simulink model "CACC_4_Robots_Example_Cases"  (R2021a)
settings: Solver=FixedStepAuto  StartTime=0.0  StopTime=Tsim  RelTol=1e-3
values from neighbouring files (symbols this model uses):
  cIN = 0    [ros_cacc.m]    (also in ros_cacc2.m = 4)
  h = 1.0    (= 1)    [ros_cacc.m]    (also in ros_cacc2.m)
  k1 = 1    [ros_cacc.m]    (also in ros_cacc2.m)
  k2 = 1    [ros_cacc.m]    (also in ros_cacc2.m)
  r = 1    [ros_cacc.m]    (also in ros_cacc2.m)
  v_0 = 0.5    [ros_cacc.m]    (also in ros_cacc2.m)
  v_threshold = v_thr    (= 0.1)    [ros_cacc.m]    (also in ros_cacc2.m)
undefined symbols (not defined in the file or in its folder): angular, linear, sigbuilder_block
libraries: ros2lib x23, robotcorelib x4
(part 1 of 3)
settings Model: Creator=harun  LastModifiedBy=harun
settings DataIOCC: DSMLogging=off  ReturnWorkspaceOutputs=off
settings OptimizationCC: EnhancedBackFolding=on  PassReuseOutputArgsAs=Individual arguments  ZeroExternalMemoryAtStartup=off  ZeroInternalMemoryAtStartup=off  MaxStackSize=64  OptimizeBlockOrder=speed  DifferentSizesBufferReuse=on  OptimizationCustomize=off  EfficientTunableParamExpr=on
settings DebuggingCC: ParameterTunabilityLossMsg=error
settings HardwareCC: ProdBitPerLong=64  ProdHWDeviceType=AMD->x86-64 (Linux 64)
settings SFSimCC: MATLABDynamicMemAlloc=off
settings RTWCC: SystemTargetFile=ert.tlc  HardwareBoard=Robot Operating System 2 (ROS 2)  TemplateMakefile=ert_default_tmf  Toolchain=Colcon Tools  TargetLang=C++
settings CodeAppCC: ForceParamTrailComments=on  IgnoreCustomStorageClasses=off  OperatorAnnotations=on  SimulinkDataObjDesc=on  SFDataObjDesc=on  InsertBlockDesc=on
settings ERTTargetCC: CodeInterfacePackaging=C++ class  SupportContinuousTime=on  SupportVariableSizeSignals=on  RootIOFormat=Structure reference

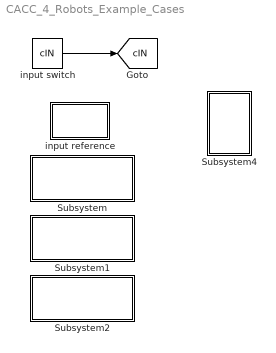
== system CACC_4_Robots_Example_Cases ==
  Subsystem : Subsystem
  Subsystem1 : Subsystem
  Subsystem2 : Subsystem
  Subsystem4 : Subsystem
  input reference : Subsystem
  input switch : Constant  Value=cIN
  tag scope: cIN=global
  wires:
  input switch/1 -> [cIN]

== system CACC_4_Robots_Example_Cases/Subsystem ==
  Bus Creator : BusCreator  Inputs=2
  Terminator : Terminator
  Terminator1 : Terminator
  To Workspace : ToWorkspace  VariableName=robot1  SaveFormat=Timeseries  SampleTime=-1
  To Workspace1 : ToWorkspace  VariableName=robot1input  SaveFormat=Timeseries  SampleTime=0.01
  controllers : Subsystem
  subscriber : Subsystem
  vehicle w/o CACC : Subsystem
  wires:
  controllers/2(z) -> Terminator/1
  vehicle w/o CACC/1(state) -> Bus Creator/1, controllers/2(state)
  controllers/1(a,w) -> vehicle w/o CACC/1(a,w)
  controllers/3(xLA,yLA) -> Bus Creator/2, Terminator1/1
  Bus Creator/1 -> To Workspace/1
  subscriber/1(state) -> To Workspace1/1, vehicle w/o CACC/2(v), controllers/1(state_prec)

== system CACC_4_Robots_Example_Cases/Subsystem1 ==
  Bus Creator : BusCreator  Inputs=2
  Terminator : Terminator
  Terminator1 : Terminator
  To Workspace : ToWorkspace  VariableName=robot2  SaveFormat=Timeseries  SampleTime=-1
  controllers : Subsystem
  subscriber : Subsystem
  vehicle w/o CACC : Subsystem
  wires:
  subscriber/1(state1) -> vehicle w/o CACC/2(v), controllers/1(state_prec)
  controllers/2(z) -> Terminator/1
  controllers/1(a,w) -> vehicle w/o CACC/1(a,w)
  vehicle w/o CACC/1(state) -> Bus Creator/1, controllers/2(state)
  controllers/3(xLA,yLA) -> Bus Creator/2, Terminator1/1
  Bus Creator/1 -> To Workspace/1

== system CACC_4_Robots_Example_Cases/Subsystem2 ==
  Bus Creator : BusCreator  Inputs=2
  Terminator : Terminator
  Terminator1 : Terminator
  To Workspace : ToWorkspace  VariableName=robot3  SaveFormat=Timeseries  SampleTime=-1
  controllers : Subsystem
  subscriber : Subsystem
  vehicle w/o CACC : Subsystem
  wires:
  subscriber/1(state) -> vehicle w/o CACC/2(v), controllers/1(state_prec)
  controllers/2(z) -> Terminator/1
  controllers/1(a,w) -> vehicle w/o CACC/1(a,w)
  vehicle w/o CACC/1(state) -> Bus Creator/1, controllers/2(state)
  controllers/3(xLA,yLA) -> Bus Creator/2, Terminator1/1
  Bus Creator/1 -> To Workspace/1

== system CACC_4_Robots_Example_Cases/Subsystem4 ==
  Subsystem3 : Subsystem
  To Workspace : ToWorkspace  VariableName=robot0  SaveFormat=Timeseries  SampleTime=-1
  wires:
  Subsystem3/1(state) -> To Workspace/1

== system CACC_4_Robots_Example_Cases/input reference ==
  Switch Case : SwitchCase  CaseConditions={1,2,3}  ShowDefaultCase=off
  circular path small curv : Subsystem  TreatAsAtomicUnit=on
  "circular path, varying velocity" : Subsystem  TreatAsAtomicUnit=on
  random path : Subsystem  TreatAsAtomicUnit=on
  wires:
  Switch Case/2 -> "circular path, varying velocity"/Action
  Switch Case/1 -> circular path small curv/Action
  [cIN] -> Switch Case/1
  Switch Case/3 -> random path/Action

== system CACC_4_Robots_Example_Cases/Subsystem/controllers ==
  state_prec : Inport
  state : Inport  Port=2
  Switch Case Ext. LA : Subsystem  TreatAsAtomicUnit=on
  a,w : Outport  VectorParamsAs1DForOutWhenUnconnected=off
  z : Outport  Port=2  VectorParamsAs1DForOutWhenUnconnected=off
  xLA,yLA : Outport  Port=3  VectorParamsAs1DForOutWhenUnconnected=off
  wires:
  state_prec/1 -> Switch Case Ext. LA/1(state_prec)
  state/1 -> Switch Case Ext. LA/2(state)
  Switch Case Ext. LA/1(a,w) -> a,w/1
  Switch Case Ext. LA/2(z) -> z/1
  Switch Case Ext. LA/3(lookahead point) -> xLA,yLA/1

== system CACC_4_Robots_Example_Cases/Subsystem/subscriber ==
  Bus Creator : BusCreator  Inputs=7
  Bus Selector : BusSelector  OutputSignals=x,y,v,vdot,theta,thetadot
  Derivative2 : Derivative
  Divide : Product  Inputs=*/
  One : Constant  OutDataTypeStr=Inherit: Inherit via back propagation
  Subscribe : ros2lib/Subscribe  topicSource=Specify your own  topic=/robot1/caccCam  messageType=ros_its_msgs/CAM  sampleTime=0.1  QOSHistory=Keep last  QOSDepth=1  QOSReliability=Reliable  QOSDurability=Volatile
      settings: SourceProductBaseCode=RR
  Switch : Switch  Criteria=u2 ~= 0
  Terminator : Terminator
  Terminator4 : Terminator
  state : Outport  VectorParamsAs1DForOutWhenUnconnected=off
  wires:
  Subscribe/1 -> Terminator/1
  Subscribe/2 -> Bus Selector/1
  Bus Selector/4 -> Terminator4/1  "<vdot>"
  One/1 -> Switch/3
  Bus Selector/1 -> Bus Creator/1  "<x>"
  Bus Selector/2 -> Bus Creator/2  "<y>"
  Derivative2/1 -> Bus Creator/4  "vdot"
  Bus Selector/5 -> Bus Creator/5  "<theta>"
  Divide/1 -> Bus Creator/7  "curv"
  Bus Selector/3 -> Bus Creator/3, Derivative2/1, Switch/2, Switch/1  "<v>"
  Bus Creator/1 -> state/1
  Switch/1 -> Divide/2
  Bus Selector/6 -> Divide/1, Bus Creator/6  "<thetadot>"

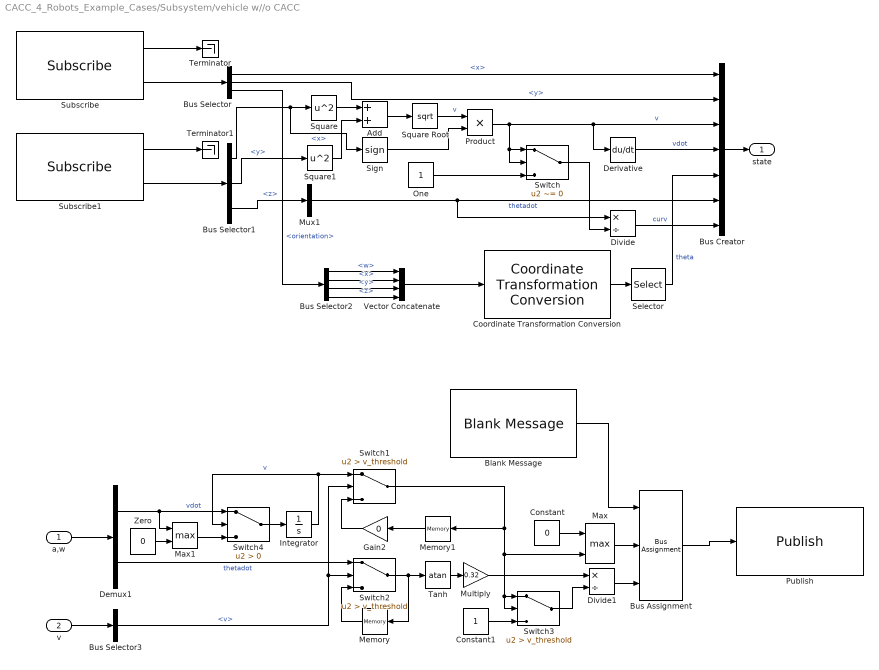
== system CACC_4_Robots_Example_Cases/Subsystem/vehicle w//o CACC ==
  a,w : Inport
  v : Inport  Port=2
  Add : Sum
  Blank Message : ros2lib/Blank Message  messageType=geometry_msgs/Twist  SampleTime=0.01
      settings: SourceProductBaseCode=RR
  Bus Assignment : BusAssignment  AssignedSignals=linear.x,angular.z
  Bus Creator : BusCreator  Inputs=7
  Bus Selector : BusSelector  OutputSignals=pose.position.x,pose.position.y,pose.orientation
  Bus Selector1 : BusSelector  OutputSignals=twist.twist.linear.x,twist.twist.linear.y,twist.twist.angular.z
  Bus Selector2 : BusSelector  OutputSignals=w,x,y,z
  Bus Selector3 : BusSelector  OutputSignals=v
  Constant : Constant  Value=0
  Constant1 : Constant
  Coordinate Transformation Conversion : robotcorelib/Coordinate Transformation Conversion  InputRepresentation=Quaternion  InputEulerSequence=ZYX  ShowTrVecInputPort=on  OutputRepresentation=Euler Angles  OutputEulerSequence=ZYX  ShowTrVecOutputPort=on  SimulateUsing=Interpreted execution
      settings: SourceProductBaseCode=NV,RO,RR,UV
  Demux1 : Demux  Outputs=2
  Derivative : Derivative
  Divide : Product  Inputs=*/
  Divide1 : Product  Inputs=*/
  Gain2 : Gain  Gain=0
  Integrator : Integrator  InitialCondition=v_0
  Max : MinMax  Function=max  Inputs=2
  Max1 : MinMax  Function=max  Inputs=2
  Memory : Memory
  Memory1 : Memory
  Multiply : Gain  Gain=0.32
  Mux1 : Mux  Inputs=1
  One : Constant  OutDataTypeStr=Inherit: Inherit via back propagation
  Product : Product
  Publish : ros2lib/Publish  topicSource=Specify your own  topic=/robot1/cmd_vel  messageType=geometry_msgs/Twist  QOSHistory=Keep last  QOSDepth=1  QOSReliability=Reliable  QOSDurability=Volatile
      settings: SourceProductBaseCode=RR
  Selector : Selector  InputPortWidth=3  IndexOptions=Index vector (dialog)  Indices=[1]  OutputSizes=1
  Sign : Signum
  Square : Math  Operator=square  SaturateOnIntegerOverflow=on
  Square Root : Sqrt  SaturateOnIntegerOverflow=on
  Square1 : Math  Operator=square  SaturateOnIntegerOverflow=on
  Subscribe : ros2lib/Subscribe  topicSource=Specify your own  topic=/robot1/robot_pose  messageType=geometry_msgs/PoseStamped  sampleTime=0.01  QOSHistory=Keep last  QOSDepth=1  QOSReliability=Reliable  QOSDurability=Volatile
      settings: SourceProductBaseCode=RR
  Subscribe1 : ros2lib/Subscribe  topicSource=Specify your own  topic=/robot1/odom  messageType=nav_msgs/Odometry  sampleTime=0.01  QOSHistory=Keep last  QOSDepth=1  QOSReliability=Reliable  QOSDurability=Volatile
      settings: SourceProductBaseCode=RR
  Switch : Switch  Criteria=u2 ~= 0
  Switch1 : Switch  Criteria=u2 > Threshold  Threshold=v_threshold
  Switch2 : Switch  Criteria=u2 > Threshold  Threshold=v_threshold
  Switch3 : Switch  Criteria=u2 > Threshold  Threshold=v_threshold
  Switch4 : Switch  Criteria=u2 > Threshold
  Tanh : Trigonometry  Operator=atan
  Terminator : Terminator
  Terminator1 : Terminator
  Vector Concatenate : Concatenate  NumInputs=4
  Zero : Constant  Value=0  OutDataTypeStr=Inherit: Inherit via back propagation
  state : Outport  VectorParamsAs1DForOutWhenUnconnected=off
  wires:
  Zero/1 -> Max1/2
  Add/1 -> Square Root/1
  Subscribe/1 -> Terminator/1
  Bus Selector1/1 -> Sign/1, Square/1  "<x>"
  a,w/1 -> Demux1/1
  Switch2/1 -> Memory/1, Tanh/1
  Constant/1 -> Max/1
  Bus Selector/2 -> Bus Creator/2  "<y>"
  Bus Selector3/1 -> Switch2/2, Switch1/2  "<v>"
  Bus Selector2/3 -> Vector Concatenate/3  "<y>"
  Bus Assignment/1 -> Publish/1
  Mux1/1 -> Divide/1, Bus Creator/6  "thetadot"
  Memory1/1 -> Gain2/1
  Switch/1 -> Divide/2
  Bus Creator/1 -> state/1
  Tanh/1 -> Multiply/1
  Subscribe1/1 -> Terminator1/1
  Max/1 -> Bus Assignment/2
  Demux1/2 -> Switch2/1  "thetadot"
  Product/1 -> Switch/1, Switch/2, Derivative/1, Bus Creator/3  "v"
  Sign/1 -> Product/2
  Bus Selector2/2 -> Vector Concatenate/2  "<x>"
  Subscribe/2 -> Bus Selector/1
  Selector/1 -> Bus Creator/5  "theta"
  Divide1/1 -> Bus Assignment/3
  Subscribe1/2 -> Bus Selector1/1
  Square1/1 -> Add/2
  Max1/1 -> Switch4/3
  v/1 -> Bus Selector3/1
  Switch1/1 -> Switch3/2, Switch3/1, Max/2, Memory1/1
  Constant1/1 -> Switch3/3
  Bus Selector1/3 -> Mux1/1  "<z>"
  Bus Selector/1 -> Bus Creator/1  "<x>"
  Divide/1 -> Bus Creator/7  "curv"
  Vector Concatenate/1 -> Coordinate Transformation Conversion/1
  Multiply/1 -> Divide1/1
  Bus Selector1/2 -> Square1/1  "<y>"
  Blank Message/1 -> Bus Assignment/1
  Derivative/1 -> Bus Creator/4  "vdot"
  Integrator/1 -> Switch4/2, Switch1/1  "v"
  Demux1/1 -> Max1/1, Switch4/1  "vdot"
  Square Root/1 -> Product/1  "v"
  Switch3/1 -> Divide1/2
  Coordinate Transformation Conversion/1 -> Selector/1
  Square/1 -> Add/1
  One/1 -> Switch/3
  Switch4/1 -> Integrator/1
  Bus Selector/3 -> Bus Selector2/1  "<orientation>"
  Bus Selector2/4 -> Vector Concatenate/4  "<z>"
  Bus Selector2/1 -> Vector Concatenate/1  "<w>"
  Gain2/1 -> Switch1/3
  Memory/1 -> Switch2/3

== system CACC_4_Robots_Example_Cases/Subsystem1/controllers ==
  state_prec : Inport
  state : Inport  Port=2
  Switch Case Ext. LA : Subsystem  TreatAsAtomicUnit=on
  a,w : Outport  VectorParamsAs1DForOutWhenUnconnected=off
  z : Outport  Port=2  VectorParamsAs1DForOutWhenUnconnected=off
  xLA,yLA : Outport  Port=3  VectorParamsAs1DForOutWhenUnconnected=off
  wires:
  state_prec/1 -> Switch Case Ext. LA/1(state_prec)
  state/1 -> Switch Case Ext. LA/2(state)
  Switch Case Ext. LA/1(a,w) -> a,w/1
  Switch Case Ext. LA/2(z) -> z/1
  Switch Case Ext. LA/3(lookahead point) -> xLA,yLA/1

== system CACC_4_Robots_Example_Cases/Subsystem1/subscriber ==
  Bus Creator1 : BusCreator  Inputs=7
  Bus Selector1 : BusSelector  OutputSignals=x,y,v,vdot,theta,thetadot
  Derivative2 : Derivative
  Divide1 : Product  Inputs=*/
  One1 : Constant  OutDataTypeStr=Inherit: Inherit via back propagation
  Subscribe : ros2lib/Subscribe  topicSource=Specify your own  topic=/robot2/caccCam  messageType=ros_its_msgs/CAM  sampleTime=0.1  QOSHistory=Keep last  QOSDepth=1  QOSReliability=Reliable  QOSDurability=Volatile
      settings: SourceProductBaseCode=RR
  Switch1 : Switch  Criteria=u2 ~= 0
  Terminator : Terminator
  Terminator4 : Terminator
  state1 : Outport  VectorParamsAs1DForOutWhenUnconnected=off
  wires:
  Subscribe/1 -> Terminator/1
  Subscribe/2 -> Bus Selector1/1
  Bus Selector1/4 -> Terminator4/1  "<vdot>"
  One1/1 -> Switch1/3
  Bus Selector1/1 -> Bus Creator1/1  "<x>"
  Bus Selector1/2 -> Bus Creator1/2  "<y>"
  Derivative2/1 -> Bus Creator1/4  "vdot"
  Bus Selector1/5 -> Bus Creator1/5  "<theta>"
  Divide1/1 -> Bus Creator1/7  "curv"
  Bus Selector1/3 -> Bus Creator1/3, Derivative2/1, Switch1/2, Switch1/1  "<v>"
  Bus Creator1/1 -> state1/1
  Switch1/1 -> Divide1/2
  Bus Selector1/6 -> Divide1/1, Bus Creator1/6  "<thetadot>"

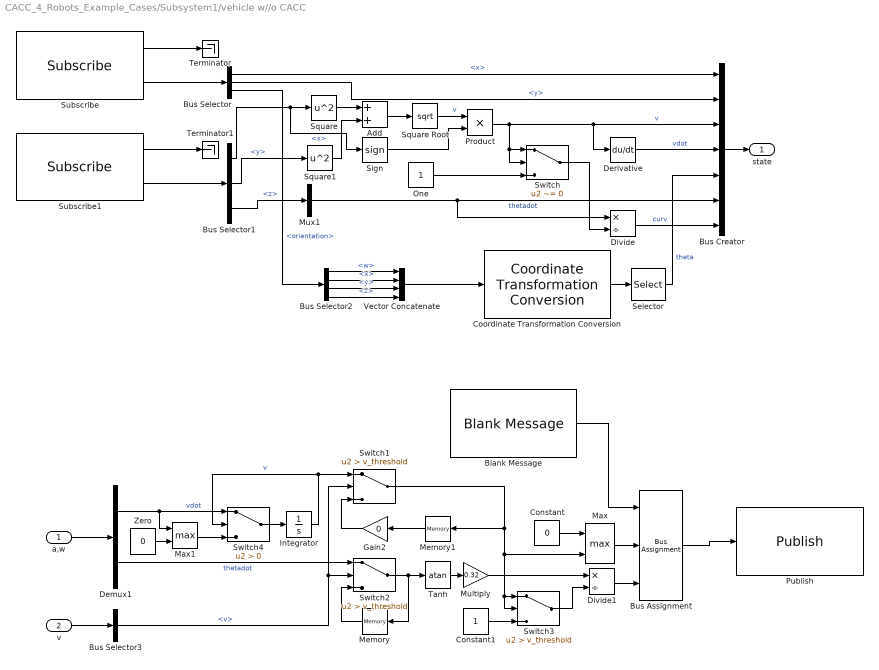
== system CACC_4_Robots_Example_Cases/Subsystem1/vehicle w//o CACC ==
  a,w : Inport
  v : Inport  Port=2
  Add : Sum
  Blank Message : ros2lib/Blank Message  messageType=geometry_msgs/Twist  SampleTime=0.01
      settings: SourceProductBaseCode=RR
  Bus Assignment : BusAssignment  AssignedSignals=linear.x,angular.z
  Bus Creator : BusCreator  Inputs=7
  Bus Selector : BusSelector  OutputSignals=pose.position.x,pose.position.y,pose.orientation
  Bus Selector1 : BusSelector  OutputSignals=twist.twist.linear.x,twist.twist.linear.y,twist.twist.angular.z
  Bus Selector2 : BusSelector  OutputSignals=w,x,y,z
  Bus Selector3 : BusSelector  OutputSignals=v
  Constant : Constant  Value=0
  Constant1 : Constant
  Coordinate Transformation Conversion : robotcorelib/Coordinate Transformation Conversion  InputRepresentation=Quaternion  InputEulerSequence=ZYX  ShowTrVecInputPort=on  OutputRepresentation=Euler Angles  OutputEulerSequence=ZYX  ShowTrVecOutputPort=on  SimulateUsing=Interpreted execution
      settings: SourceProductBaseCode=NV,RO,RR,UV
  Demux1 : Demux  Outputs=2
  Derivative : Derivative
  Divide : Product  Inputs=*/
  Divide1 : Product  Inputs=*/
  Gain2 : Gain  Gain=0
  Integrator : Integrator  InitialCondition=v_0
  Max : MinMax  Function=max  Inputs=2
  Max1 : MinMax  Function=max  Inputs=2
  Memory : Memory
  Memory1 : Memory
  Multiply : Gain  Gain=0.32
  Mux1 : Mux  Inputs=1
  One : Constant  OutDataTypeStr=Inherit: Inherit via back propagation
  Product : Product
  Publish : ros2lib/Publish  topicSource=Specify your own  topic=/robot2/cmd_vel  messageType=geometry_msgs/Twist  QOSHistory=Keep last  QOSDepth=1  QOSReliability=Reliable  QOSDurability=Volatile
      settings: SourceProductBaseCode=RR
  Selector : Selector  InputPortWidth=3  IndexOptions=Index vector (dialog)  Indices=[1]  OutputSizes=1
  Sign : Signum
  Square : Math  Operator=square  SaturateOnIntegerOverflow=on
  Square Root : Sqrt  SaturateOnIntegerOverflow=on
  Square1 : Math  Operator=square  SaturateOnIntegerOverflow=on
  Subscribe : ros2lib/Subscribe  topicSource=Specify your own  topic=/robot2/robot_pose  messageType=geometry_msgs/PoseStamped  sampleTime=0.01  QOSHistory=Keep last  QOSDepth=1  QOSReliability=Reliable  QOSDurability=Volatile
      settings: SourceProductBaseCode=RR
  Subscribe1 : ros2lib/Subscribe  topicSource=Specify your own  topic=/robot2/odom  messageType=nav_msgs/Odometry  sampleTime=0.01  QOSHistory=Keep last  QOSDepth=1  QOSReliability=Reliable  QOSDurability=Volatile
      settings: SourceProductBaseCode=RR
  Switch : Switch  Criteria=u2 ~= 0
  Switch1 : Switch  Criteria=u2 > Threshold  Threshold=v_threshold
  Switch2 : Switch  Criteria=u2 > Threshold  Threshold=v_threshold
  Switch3 : Switch  Criteria=u2 > Threshold  Threshold=v_threshold
  Switch4 : Switch  Criteria=u2 > Threshold
  Tanh : Trigonometry  Operator=atan
  Terminator : Terminator
  Terminator1 : Terminator
  Vector Concatenate : Concatenate  NumInputs=4
  Zero : Constant  Value=0  OutDataTypeStr=Inherit: Inherit via back propagation
  state : Outport  VectorParamsAs1DForOutWhenUnconnected=off
  wires:
  Zero/1 -> Max1/2
  Add/1 -> Square Root/1
  Subscribe/1 -> Terminator/1
  Bus Selector1/1 -> Sign/1, Square/1  "<x>"
  a,w/1 -> Demux1/1
  Switch2/1 -> Memory/1, Tanh/1
  Constant/1 -> Max/1
  Bus Selector/2 -> Bus Creator/2  "<y>"
  Bus Selector3/1 -> Switch2/2, Switch1/2  "<v>"
  Bus Selector2/3 -> Vector Concatenate/3  "<y>"
  Bus Assignment/1 -> Publish/1
  Mux1/1 -> Divide/1, Bus Creator/6  "thetadot"
  Memory1/1 -> Gain2/1
  Switch/1 -> Divide/2
  Bus Creator/1 -> state/1
  Tanh/1 -> Multiply/1
  Subscribe1/1 -> Terminator1/1
  Max/1 -> Bus Assignment/2
  Demux1/2 -> Switch2/1  "thetadot"
  Product/1 -> Switch/1, Switch/2, Derivative/1, Bus Creator/3  "v"
  Sign/1 -> Product/2
  Bus Selector2/2 -> Vector Concatenate/2  "<x>"
  Subscribe/2 -> Bus Selector/1
  Selector/1 -> Bus Creator/5  "theta"
  Divide1/1 -> Bus Assignment/3
  Subscribe1/2 -> Bus Selector1/1
  Square1/1 -> Add/2
  Max1/1 -> Switch4/3
  v/1 -> Bus Selector3/1
  Switch1/1 -> Switch3/2, Switch3/1, Max/2, Memory1/1
  Constant1/1 -> Switch3/3
  Bus Selector1/3 -> Mux1/1  "<z>"
  Bus Selector/1 -> Bus Creator/1  "<x>"
  Divide/1 -> Bus Creator/7  "curv"
  Vector Concatenate/1 -> Coordinate Transformation Conversion/1
  Multiply/1 -> Divide1/1
  Bus Selector1/2 -> Square1/1  "<y>"
  Blank Message/1 -> Bus Assignment/1
  Derivative/1 -> Bus Creator/4  "vdot"
  Integrator/1 -> Switch4/2, Switch1/1  "v"
  Demux1/1 -> Max1/1, Switch4/1  "vdot"
  Square Root/1 -> Product/1  "v"
  Switch3/1 -> Divide1/2
  Coordinate Transformation Conversion/1 -> Selector/1
  Square/1 -> Add/1
  One/1 -> Switch/3
  Switch4/1 -> Integrator/1
  Bus Selector/3 -> Bus Selector2/1  "<orientation>"
  Bus Selector2/4 -> Vector Concatenate/4  "<z>"
  Bus Selector2/1 -> Vector Concatenate/1  "<w>"
  Gain2/1 -> Switch1/3
  Memory/1 -> Switch2/3

== system CACC_4_Robots_Example_Cases/Subsystem2/controllers ==
  state_prec : Inport
  state : Inport  Port=2
  Switch Case Ext. LA : Subsystem  TreatAsAtomicUnit=on
  a,w : Outport  VectorParamsAs1DForOutWhenUnconnected=off
  z : Outport  Port=2  VectorParamsAs1DForOutWhenUnconnected=off
  xLA,yLA : Outport  Port=3  VectorParamsAs1DForOutWhenUnconnected=off
  wires:
  state_prec/1 -> Switch Case Ext. LA/1(state_prec)
  state/1 -> Switch Case Ext. LA/2(state)
  Switch Case Ext. LA/1(a,w) -> a,w/1
  Switch Case Ext. LA/2(z) -> z/1
  Switch Case Ext. LA/3(lookahead point) -> xLA,yLA/1

== system CACC_4_Robots_Example_Cases/Subsystem2/subscriber ==
  Bus Creator : BusCreator  Inputs=7
  Bus Selector : BusSelector  OutputSignals=x,y,v,vdot,theta,thetadot
  Derivative2 : Derivative
  Divide : Product  Inputs=*/
  One : Constant  OutDataTypeStr=Inherit: Inherit via back propagation
  Subscribe : ros2lib/Subscribe  topicSource=Specify your own  topic=/robot3/caccCam  messageType=ros_its_msgs/CAM  sampleTime=0.1  QOSHistory=Keep last  QOSDepth=1  QOSReliability=Reliable  QOSDurability=Volatile
      settings: SourceProductBaseCode=RR
  Switch : Switch  Criteria=u2 ~= 0
  Terminator : Terminator
  Terminator4 : Terminator
  state : Outport  VectorParamsAs1DForOutWhenUnconnected=off
  wires:
  Subscribe/1 -> Terminator/1
  Subscribe/2 -> Bus Selector/1
  Bus Selector/4 -> Terminator4/1  "<vdot>"
  One/1 -> Switch/3
  Bus Selector/1 -> Bus Creator/1  "<x>"
  Bus Selector/2 -> Bus Creator/2  "<y>"
  Derivative2/1 -> Bus Creator/4  "vdot"
  Bus Selector/5 -> Bus Creator/5  "<theta>"
  Divide/1 -> Bus Creator/7  "curv"
  Bus Selector/3 -> Bus Creator/3, Derivative2/1, Switch/2, Switch/1  "<v>"
  Bus Creator/1 -> state/1
  Switch/1 -> Divide/2
  Bus Selector/6 -> Divide/1, Bus Creator/6  "<thetadot>"

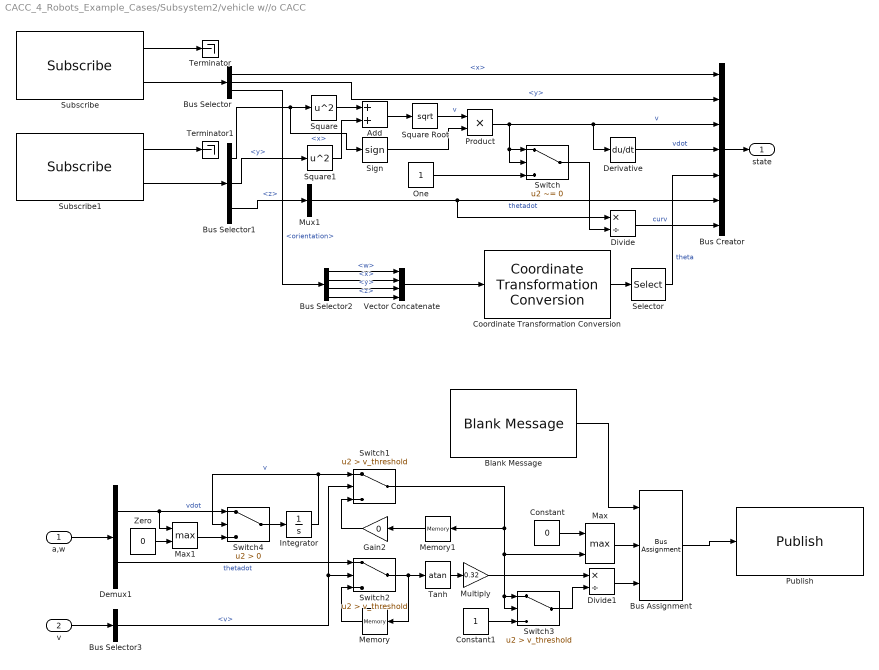
== system CACC_4_Robots_Example_Cases/Subsystem2/vehicle w//o CACC ==
  a,w : Inport
  v : Inport  Port=2
  Add : Sum
  Blank Message : ros2lib/Blank Message  messageType=geometry_msgs/Twist  SampleTime=0.01
      settings: SourceProductBaseCode=RR
  Bus Assignment : BusAssignment  AssignedSignals=linear.x,angular.z
  Bus Creator : BusCreator  Inputs=7
  Bus Selector : BusSelector  OutputSignals=pose.position.x,pose.position.y,pose.orientation
  Bus Selector1 : BusSelector  OutputSignals=twist.twist.linear.x,twist.twist.linear.y,twist.twist.angular.z
  Bus Selector2 : BusSelector  OutputSignals=w,x,y,z
  Bus Selector3 : BusSelector  OutputSignals=v
  Constant : Constant  Value=0
  Constant1 : Constant
  Coordinate Transformation Conversion : robotcorelib/Coordinate Transformation Conversion  InputRepresentation=Quaternion  InputEulerSequence=ZYX  ShowTrVecInputPort=on  OutputRepresentation=Euler Angles  OutputEulerSequence=ZYX  ShowTrVecOutputPort=on  SimulateUsing=Interpreted execution
      settings: SourceProductBaseCode=NV,RO,RR,UV
  Demux1 : Demux  Outputs=2
  Derivative : Derivative
  Divide : Product  Inputs=*/
  Divide1 : Product  Inputs=*/
  Gain2 : Gain  Gain=0
  Integrator : Integrator  InitialCondition=v_0
  Max : MinMax  Function=max  Inputs=2
  Max1 : MinMax  Function=max  Inputs=2
  Memory : Memory
  Memory1 : Memory
  Multiply : Gain  Gain=0.32
  Mux1 : Mux  Inputs=1
  One : Constant  OutDataTypeStr=Inherit: Inherit via back propagation
  Product : Product
  Publish : ros2lib/Publish  topicSource=Specify your own  topic=/robot3/cmd_vel  messageType=geometry_msgs/Twist  QOSHistory=Keep last  QOSDepth=1  QOSReliability=Reliable  QOSDurability=Volatile
      settings: SourceProductBaseCode=RR
  Selector : Selector  InputPortWidth=3  IndexOptions=Index vector (dialog)  Indices=[1]  OutputSizes=1
  Sign : Signum
  Square : Math  Operator=square  SaturateOnIntegerOverflow=on
  Square Root : Sqrt  SaturateOnIntegerOverflow=on
  Square1 : Math  Operator=square  SaturateOnIntegerOverflow=on
  Subscribe : ros2lib/Subscribe  topicSource=Specify your own  topic=/robot3/robot_pose  messageType=geometry_msgs/PoseStamped  sampleTime=0.01  QOSHistory=Keep last  QOSDepth=1  QOSReliability=Reliable  QOSDurability=Volatile
      settings: SourceProductBaseCode=RR
  Subscribe1 : ros2lib/Subscribe  topicSource=Specify your own  topic=/robot3/odom  messageType=nav_msgs/Odometry  sampleTime=0.01  QOSHistory=Keep last  QOSDepth=1  QOSReliability=Reliable  QOSDurability=Volatile
      settings: SourceProductBaseCode=RR
  Switch : Switch  Criteria=u2 ~= 0
  Switch1 : Switch  Criteria=u2 > Threshold  Threshold=v_threshold
  Switch2 : Switch  Criteria=u2 > Threshold  Threshold=v_threshold
  Switch3 : Switch  Criteria=u2 > Threshold  Threshold=v_threshold
  Switch4 : Switch  Criteria=u2 > Threshold
  Tanh : Trigonometry  Operator=atan
  Terminator : Terminator
  Terminator1 : Terminator
  Vector Concatenate : Concatenate  NumInputs=4
  Zero : Constant  Value=0  OutDataTypeStr=Inherit: Inherit via back propagation
  state : Outport  VectorParamsAs1DForOutWhenUnconnected=off
  wires:
  Zero/1 -> Max1/2
  Add/1 -> Square Root/1
  Subscribe/1 -> Terminator/1
  Bus Selector1/1 -> Sign/1, Square/1  "<x>"
  a,w/1 -> Demux1/1
  Switch2/1 -> Memory/1, Tanh/1
  Constant/1 -> Max/1
  Bus Selector/2 -> Bus Creator/2  "<y>"
  Bus Selector3/1 -> Switch2/2, Switch1/2  "<v>"
  Bus Selector2/3 -> Vector Concatenate/3  "<y>"
  Bus Assignment/1 -> Publish/1
  Mux1/1 -> Divide/1, Bus Creator/6  "thetadot"
  Memory1/1 -> Gain2/1
  Switch/1 -> Divide/2
  Bus Creator/1 -> state/1
  Tanh/1 -> Multiply/1
  Subscribe1/1 -> Terminator1/1
  Max/1 -> Bus Assignment/2
  Demux1/2 -> Switch2/1  "thetadot"
  Product/1 -> Switch/1, Switch/2, Derivative/1, Bus Creator/3  "v"
  Sign/1 -> Product/2
  Bus Selector2/2 -> Vector Concatenate/2  "<x>"
  Subscribe/2 -> Bus Selector/1
  Selector/1 -> Bus Creator/5  "theta"
  Divide1/1 -> Bus Assignment/3
  Subscribe1/2 -> Bus Selector1/1
  Square1/1 -> Add/2
  Max1/1 -> Switch4/3
  v/1 -> Bus Selector3/1
  Switch1/1 -> Switch3/2, Switch3/1, Max/2, Memory1/1
  Constant1/1 -> Switch3/3
  Bus Selector1/3 -> Mux1/1  "<z>"
  Bus Selector/1 -> Bus Creator/1  "<x>"
  Divide/1 -> Bus Creator/7  "curv"
  Vector Concatenate/1 -> Coordinate Transformation Conversion/1
  Multiply/1 -> Divide1/1
  Bus Selector1/2 -> Square1/1  "<y>"
  Blank Message/1 -> Bus Assignment/1
  Derivative/1 -> Bus Creator/4  "vdot"
  Integrator/1 -> Switch4/2, Switch1/1  "v"
  Demux1/1 -> Max1/1, Switch4/1  "vdot"
  Square Root/1 -> Product/1  "v"
  Switch3/1 -> Divide1/2
  Coordinate Transformation Conversion/1 -> Selector/1
  Square/1 -> Add/1
  One/1 -> Switch/3
  Switch4/1 -> Integrator/1
  Bus Selector/3 -> Bus Selector2/1  "<orientation>"
  Bus Selector2/4 -> Vector Concatenate/4  "<z>"
  Bus Selector2/1 -> Vector Concatenate/1  "<w>"
  Gain2/1 -> Switch1/3
  Memory/1 -> Switch2/3

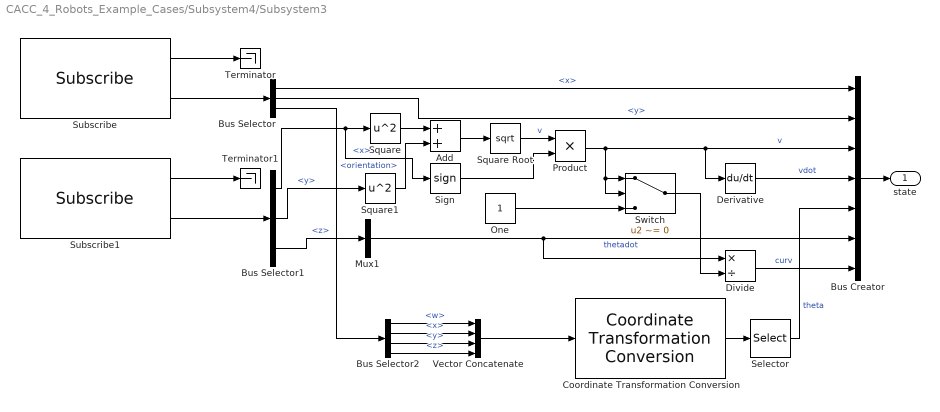
== system CACC_4_Robots_Example_Cases/Subsystem4/Subsystem3 ==
  Add : Sum
  Bus Creator : BusCreator  Inputs=7
  Bus Selector : BusSelector  OutputSignals=pose.position.x,pose.position.y,pose.orientation
  Bus Selector1 : BusSelector  OutputSignals=twist.twist.linear.x,twist.twist.linear.y,twist.twist.angular.z
  Bus Selector2 : BusSelector  OutputSignals=w,x,y,z
  Coordinate Transformation Conversion : robotcorelib/Coordinate Transformation Conversion  InputRepresentation=Quaternion  InputEulerSequence=ZYX  ShowTrVecInputPort=on  OutputRepresentation=Euler Angles  OutputEulerSequence=ZYX  ShowTrVecOutputPort=on  SimulateUsing=Interpreted execution
      settings: SourceProductBaseCode=NV,RO,RR,UV
  Derivative : Derivative
  Divide : Product  Inputs=*/
  Mux1 : Mux  Inputs=1
  One : Constant  OutDataTypeStr=Inherit: Inherit via back propagation
  Product : Product
  Selector : Selector  InputPortWidth=3  IndexOptions=Index vector (dialog)  Indices=[1]  OutputSizes=1
  Sign : Signum
  Square : Math  Operator=square  SaturateOnIntegerOverflow=on
  Square Root : Sqrt  SaturateOnIntegerOverflow=on
  Square1 : Math  Operator=square  SaturateOnIntegerOverflow=on
  Subscribe : ros2lib/Subscribe  topicSource=Specify your own  topic=/robot0/robot_pose  messageType=geometry_msgs/PoseStamped  sampleTime=0.01  QOSHistory=Keep last  QOSDepth=1  QOSReliability=Reliable  QOSDurability=Volatile
      settings: SourceProductBaseCode=RR
  Subscribe1 : ros2lib/Subscribe  topicSource=Specify your own  topic=/robot0/odom  messageType=nav_msgs/Odometry  sampleTime=0.01  QOSHistory=Keep last  QOSDepth=1  QOSReliability=Reliable  QOSDurability=Volatile
      settings: SourceProductBaseCode=RR
  Switch : Switch  Criteria=u2 ~= 0
  Terminator : Terminator
  Terminator1 : Terminator
  Vector Concatenate : Concatenate  NumInputs=4
  state : Outport  VectorParamsAs1DForOutWhenUnconnected=off
  wires:
  Bus Selector/3 -> Bus Selector2/1  "<orientation>"
  Product/1 -> Switch/1, Switch/2, Derivative/1, Bus Creator/3  "v"
  Subscribe/1 -> Terminator/1
  Sign/1 -> Product/2
  Bus Selector2/3 -> Vector Concatenate/3  "<y>"
  Selector/1 -> Bus Creator/5  "theta"
  Subscribe1/1 -> Terminator1/1
  Derivative/1 -> Bus Creator/4  "vdot"
  Subscribe/2 -> Bus Selector/1
  One/1 -> Switch/3
  Bus Selector1/1 -> Sign/1, Square/1  "<x>"
  Bus Creator/1 -> state/1
  Square/1 -> Add/1
  Bus Selector/2 -> Bus Creator/2  "<y>"
  Bus Selector1/3 -> Mux1/1  "<z>"
  Switch/1 -> Divide/2
  Bus Selector/1 -> Bus Creator/1  "<x>"
  Square Root/1 -> Product/1  "v"
  Square1/1 -> Add/2
  Coordinate Transformation Conversion/1 -> Selector/1
  Bus Selector2/2 -> Vector Concatenate/2  "<x>"
  Divide/1 -> Bus Creator/7  "curv"
  Bus Selector2/1 -> Vector Concatenate/1  "<w>"
  Add/1 -> Square Root/1
  Bus Selector1/2 -> Square1/1  "<y>"
  Subscribe1/2 -> Bus Selector1/1
  Vector Concatenate/1 -> Coordinate Transformation Conversion/1
  Bus Selector2/4 -> Vector Concatenate/4  "<z>"
  Mux1/1 -> Divide/1, Bus Creator/6  "thetadot"

== system CACC_4_Robots_Example_Cases/input reference/circular path small curv ==
  Action Port : ActionPort  PropagateVarSize=During execution  ActionPortLabel=case [ 1 ]:
  Blank Message2 : ros2lib/Blank Message  messageType=geometry_msgs/Twist  SampleTime=0
      settings: SourceProductBaseCode=RR
  Bus Assignment1 : BusAssignment  AssignedSignals=linear.x,angular.z
  Integrator : Integrator  InitialCondition=1
  Publish2 : ros2lib/Publish  topicSource=Specify your own  topic=/robot0/cmd_vel  messageType=geometry_msgs/Twist  QOSHistory=Keep last  QOSDepth=1  QOSReliability=Reliable  QOSDurability=Volatile
      settings: SourceProductBaseCode=RR
  signal: circular path1 : Subsystem  Tag=STV Subsys  LoadFcn=sigbuilder_block('load');  StartFcn=sigbuilder_block('start');  StopFcn=sigbuilder_block('stop');  ClipboardFcn=sigbuilder_block('clipboard');  mask(Sigbuilder block){tuvar=[0:10]}
      mask help: Simulink:masks:SigbuilderBlock_MD
      mask init:
      | if ~strcmp(get_param(bdroot(gcbh),'SimulationStatus'),'stopped') tuvar = sigbuilder_block('maskInit'); end
      settings: CopyFcn=sigbuilder_block('copy');  DeleteFcn=sigbuilder_block('delete');  ModelCloseFcn=sigbuilder_block('modelClose');  PreSaveFcn=sigbuilder_block('preSave');  PauseFcn=sigbuilder_block('pause');  ContinueFcn=sigbuilder_block('continue');  NameChangeFcn=sigbuilder_block('namechange');  OpenFcn=sigbuilder_block('open',[639 78 638.25 546.75 ]);  CloseFcn=sigbuilder_block('close');
      mask Display: plot(0, 0, 100, 100,[2, 2, 32, 32, 2], [68, 8, 8, 68, 68],[32, 2], [38, 38], [32, 19, 2],[53, 60, 44], [32, 17, 17, 2],[16, 16, 31, 31]);txt = getActiveGroup(gcbh);text(2, 100, txt,'verticalAlignment', 'top');
  wires:
  signal: circular path1/1(a) -> Integrator/1
  signal: circular path1/2(omega) -> Bus Assignment1/3
  Bus Assignment1/1 -> Publish2/1
  Blank Message2/1 -> Bus Assignment1/1
  Integrator/1 -> Bus Assignment1/2

== system CACC_4_Robots_Example_Cases/input reference/circular path, varying velocity ==
  Action Port : ActionPort  PropagateVarSize=During execution  ActionPortLabel=case [ 2 ]:
  Blank Message2 : ros2lib/Blank Message  messageType=geometry_msgs/Twist  SampleTime=0
      settings: SourceProductBaseCode=RR
  Bus Assignment1 : BusAssignment  AssignedSignals=linear.x,angular.z
  Integrator : Integrator  InitialCondition=0.5
  Publish2 : ros2lib/Publish  topicSource=Specify your own  topic=/robot0/cmd_vel  messageType=geometry_msgs/Twist  QOSHistory=Keep last  QOSDepth=1  QOSReliability=Reliable  QOSDurability=Volatile
      settings: SourceProductBaseCode=RR
  signal: circular path1 : Subsystem  Tag=STV Subsys  LoadFcn=sigbuilder_block('load');  StartFcn=sigbuilder_block('start');  StopFcn=sigbuilder_block('stop');  ClipboardFcn=sigbuilder_block('clipboard');  mask(Sigbuilder block){tuvar=[0:10]}
      mask help: Simulink:masks:SigbuilderBlock_MD
      mask init:
      | if ~strcmp(get_param(bdroot(gcbh),'SimulationStatus'),'stopped') tuvar = sigbuilder_block('maskInit'); end
      settings: CopyFcn=sigbuilder_block('copy');  DeleteFcn=sigbuilder_block('delete');  ModelCloseFcn=sigbuilder_block('modelClose');  PreSaveFcn=sigbuilder_block('preSave');  PauseFcn=sigbuilder_block('pause');  ContinueFcn=sigbuilder_block('continue');  NameChangeFcn=sigbuilder_block('namechange');  OpenFcn=sigbuilder_block('open',[558 95.25 630.75 552 ]);  CloseFcn=sigbuilder_block('close');
      mask Display: plot(0, 0, 100, 100,[2, 2, 32, 32, 2], [68, 8, 8, 68, 68],[32, 2], [38, 38], [32, 19, 2],[53, 60, 44], [32, 17, 17, 2],[16, 16, 31, 31]);txt = getActiveGroup(gcbh);text(2, 100, txt,'verticalAlignment', 'top');
  wires:
  Blank Message2/1 -> Bus Assignment1/1
  signal: circular path1/2(omega) -> Bus Assignment1/3
  signal: circular path1/1(a) -> Integrator/1
  Bus Assignment1/1 -> Publish2/1
  Integrator/1 -> Bus Assignment1/2

== system CACC_4_Robots_Example_Cases/input reference/random path ==
  Action Port : ActionPort  PropagateVarSize=During execution  ActionPortLabel=case [ 3 ]:
  Blank Message2 : ros2lib/Blank Message  messageType=geometry_msgs/Twist  SampleTime=0
      settings: SourceProductBaseCode=RR
  Bus Assignment1 : BusAssignment  AssignedSignals=linear.x,angular.z
  Integrator : Integrator  InitialCondition=1
  Publish2 : ros2lib/Publish  topicSource=Specify your own  topic=/robot0/cmd_vel  messageType=geometry_msgs/Twist  QOSHistory=Keep last  QOSDepth=1  QOSReliability=Reliable  QOSDurability=Volatile
      settings: SourceProductBaseCode=RR
  signal: lane changing : Subsystem  Tag=STV Subsys  LoadFcn=sigbuilder_block('load');  StartFcn=sigbuilder_block('start');  StopFcn=sigbuilder_block('stop');  ClipboardFcn=sigbuilder_block('clipboard');  mask(Sigbuilder block){tuvar=[0:10]}
      mask help: Simulink:masks:SigbuilderBlock_MD
      mask init:
      | if ~strcmp(get_param(bdroot(gcbh),'SimulationStatus'),'stopped') tuvar = sigbuilder_block('maskInit'); end
      settings: CopyFcn=sigbuilder_block('copy');  DeleteFcn=sigbuilder_block('delete');  ModelCloseFcn=sigbuilder_block('modelClose');  PreSaveFcn=sigbuilder_block('preSave');  PauseFcn=sigbuilder_block('pause');  ContinueFcn=sigbuilder_block('continue');  NameChangeFcn=sigbuilder_block('namechange');  OpenFcn=sigbuilder_block('open',[54 0 1866 939 ]);  CloseFcn=sigbuilder_block('close');
      mask Display: plot(0, 0, 100, 100,[2, 2, 32, 32, 2], [68, 8, 8, 68, 68],[32, 2], [38, 38], [32, 19, 2],[53, 60, 44], [32, 17, 17, 2],[16, 16, 31, 31]);txt = getActiveGroup(gcbh);text(2, 100, txt,'verticalAlignment', 'top');
  wires:
  Blank Message2/1 -> Bus Assignment1/1
  signal: lane changing/2(omega) -> Bus Assignment1/3
  signal: lane changing/1(a) -> Integrator/1
  Bus Assignment1/1 -> Publish2/1
  Integrator/1 -> Bus Assignment1/2

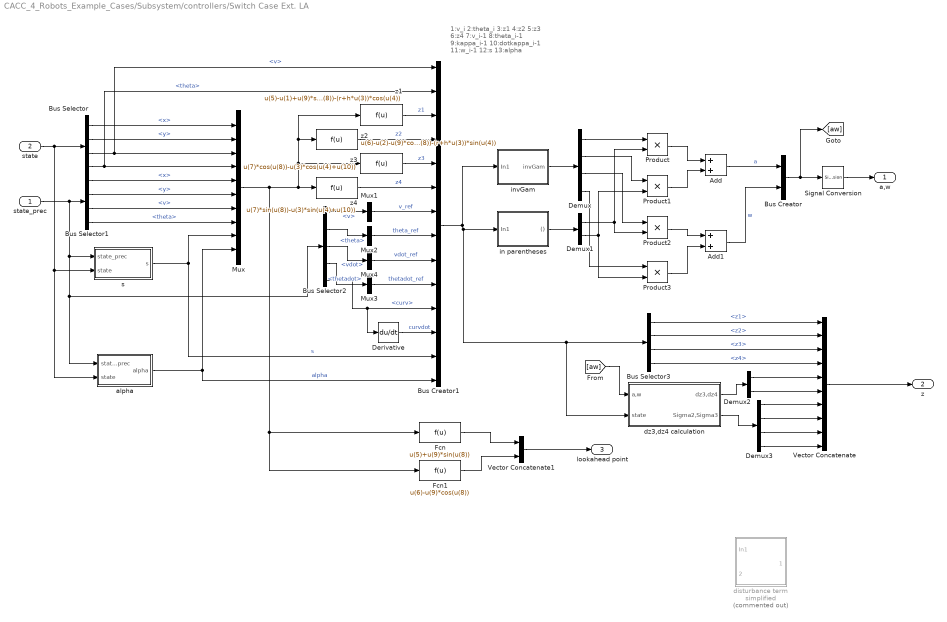
== system CACC_4_Robots_Example_Cases/Subsystem/controllers/Switch Case Ext. LA ==
  note: 1:v_i
      | 2:theta_i
      | 3:z1
      | 4:z2
      | 5:z3
      | 6:z4
      | 7:v_i-1
      | 8:theta_i-1
      | 9:kappa_i-1
      | 10:dotkappa_i-1
      | 11:w_i-1
      | 12:s
      | 13:alpha
  state_prec : Inport
  state : Inport  Port=2
  Add : Sum
  Add1 : Sum
  Bus Creator : BusCreator  Inputs=2
  Bus Creator1 : BusCreator  Inputs=14
  Bus Selector : BusSelector  OutputSignals=x,y,v,theta
  Bus Selector1 : BusSelector  OutputSignals=x,y,v,theta
  Bus Selector2 : BusSelector  OutputSignals=v,theta,vdot,thetadot,curv
  Bus Selector3 : BusSelector  OutputSignals=z1,z2,z3,z4
  Demux : Demux
  Demux1 : Demux  Outputs=2
  Demux2 : Demux  Outputs=2
  Demux3 : Demux
  Derivative : Derivative
  Fcn : Fcn  Expr=u(5)+u(9)*sin(u(8))
  Fcn1 : Fcn  Expr=u(6)-u(9)*cos(u(8))
  Mux : Mux  Inputs=10
  Mux{1..4} (4 alike) : Mux  Inputs=1
  Product{,1..3} (4 alike) : Product
  Signal Conversion : SignalConversion  OverrideOpt=off
  Vector Concatenate : Concatenate  NumInputs=10
  Vector Concatenate1 : Concatenate
  alpha : Subsystem
  disturbance term simplified : Subsystem  Commented=on
  dz3,dz4 calculation : Subsystem
  in parentheses : Subsystem
  invGam : Subsystem
  s : Subsystem
  z1 : Fcn  Expr=u(5)-u(1)+u(9)*sin(u(8))-(r+h*u(3))*cos(u(4))
  z2 : Fcn  Expr=u(6)-u(2)-u(9)*cos(u(8))-(r+h*u(3))*sin(u(4))
  z3 : Fcn  Expr=u(7)*cos(u(8))-u(3)*cos(u(4)+u(10))
  z4 : Fcn  Expr=u(7)*sin(u(8))-u(3)*sin(u(4)+u(10))
  a,w : Outport  VectorParamsAs1DForOutWhenUnconnected=off
  z : Outport  Port=2  VectorParamsAs1DForOutWhenUnconnected=off
  lookahead point : Outport  Port=3  VectorParamsAs1DForOutWhenUnconnected=off
  wires:
  Bus Selector/1 -> Mux/1  "<x>"
  Bus Selector/2 -> Mux/2  "<y>"
  Bus Selector/3 -> Bus Creator1/1, Mux/3  "<v>"
  Bus Selector/4 -> Bus Creator1/2, Mux/4  "<theta>"
  Bus Selector1/1 -> Mux/5  "<x>"
  Bus Selector1/2 -> Mux/6  "<y>"
  Bus Selector1/3 -> Mux/7  "<v>"
  Bus Selector1/4 -> Mux/8  "<theta>"
  Bus Creator/1 -> Signal Conversion/1, [aw]
  state/1 -> alpha/2(state), s/2(state), Bus Selector/1
  state_prec/1 -> alpha/1(state_prec), Bus Selector2/1, s/1(state_prec), Bus Selector1/1
  Mux/1 -> Fcn1/1, Fcn/1, z4/1, z1/1, z2/1, z3/1
  z1/1 -> Bus Creator1/3  "z1"
  z2/1 -> Bus Creator1/4  "z2"
  z3/1 -> Bus Creator1/5  "z3"
  z4/1 -> Bus Creator1/6  "z4"
  alpha/1(alpha) -> Bus Creator1/14, Mux/10  "alpha"
  s/1(s) -> Bus Creator1/13, Mux/9  "s"
  Bus Selector2/1 -> Mux1/1  "<v>"
  Bus Selector2/2 -> Mux2/1  "<theta>"
  Bus Selector2/5 -> Bus Creator1/11, Derivative/1  "<curv>"
  Derivative/1 -> Bus Creator1/12  "curvdot"
  Bus Selector2/4 -> Mux3/1  "<thetadot>"
  Bus Creator1/1 -> invGam/1(In1), dz3,dz4 calculation/2(state), Bus Selector3/1, in parentheses/1(In1)
  invGam/1(invGam) -> Demux/1
  Demux/1 -> Product/1
  in parentheses/1(()) -> Demux1/1
  Demux1/1 -> Product2/2, Product/2
  Demux/2 -> Product1/1
  Product/1 -> Add/1
  Product1/1 -> Add/2
  Demux/3 -> Product2/1
  Demux/4 -> Product3/1
  Demux1/2 -> Product1/2, Product3/2
  Product2/1 -> Add1/1
  Product3/1 -> Add1/2
  Add1/1 -> Bus Creator/2  "w"
  Mux1/1 -> Bus Creator1/7  "v_ref"
  Mux2/1 -> Bus Creator1/8  "theta_ref"
  Bus Selector3/1 -> Vector Concatenate/1  "<z1>"
  Bus Selector3/2 -> Vector Concatenate/2  "<z2>"
  Bus Selector3/3 -> Vector Concatenate/3  "<z3>"
  Bus Selector3/4 -> Vector Concatenate/4  "<z4>"
  Vector Concatenate/1 -> z/1
  Vector Concatenate1/1 -> lookahead point/1
  Fcn/1 -> Vector Concatenate1/1
  Fcn1/1 -> Vector Concatenate1/2
  dz3,dz4 calculation/1(dz3,dz4) -> Demux2/1
  [aw] -> dz3,dz4 calculation/1(a,w)
  Add/1 -> Bus Creator/1  "a"
  Demux2/1 -> Vector Concatenate/5
  Demux2/2 -> Vector Concatenate/6
  Signal Conversion/1 -> a,w/1
  Mux3/1 -> Bus Creator1/10  "thetadot_ref"
  Mux4/1 -> Bus Creator1/9  "vdot_ref"
  Bus Selector2/3 -> Mux4/1  "<vdot>"
  dz3,dz4 calculation/2(Sigma2,Sigma3) -> Demux3/1
  Demux3/1 -> Vector Concatenate/7
  Demux3/2 -> Vector Concatenate/8
  Demux3/3 -> Vector Concatenate/9
  Demux3/4 -> Vector Concatenate/10

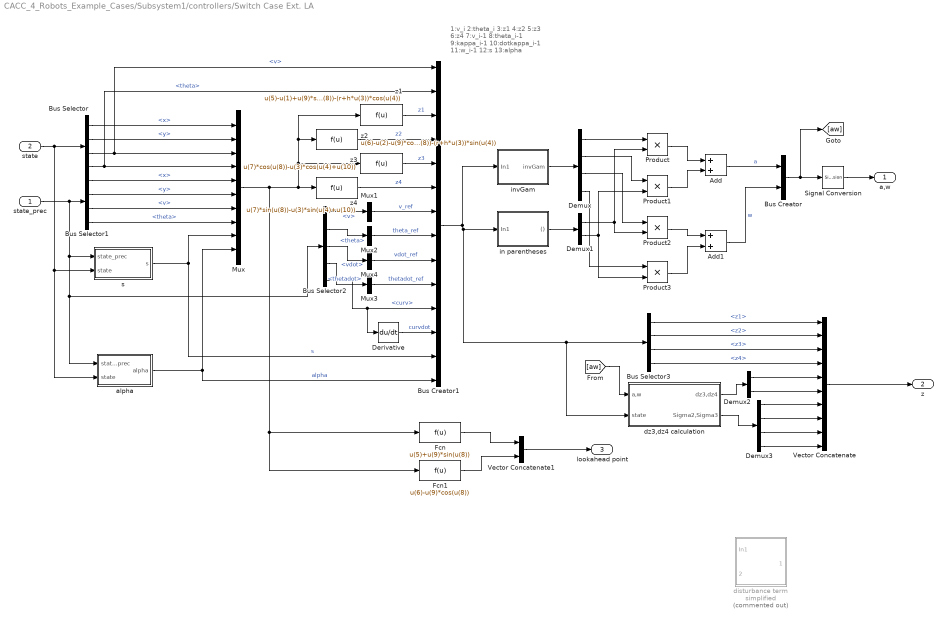
== system CACC_4_Robots_Example_Cases/Subsystem1/controllers/Switch Case Ext. LA ==
  note: 1:v_i
      | 2:theta_i
      | 3:z1
      | 4:z2
      | 5:z3
      | 6:z4
      | 7:v_i-1
      | 8:theta_i-1
      | 9:kappa_i-1
      | 10:dotkappa_i-1
      | 11:w_i-1
      | 12:s
      | 13:alpha
  state_prec : Inport
  state : Inport  Port=2
  Add : Sum
  Add1 : Sum
  Bus Creator : BusCreator  Inputs=2
  Bus Creator1 : BusCreator  Inputs=14
  Bus Selector : BusSelector  OutputSignals=x,y,v,theta
  Bus Selector1 : BusSelector  OutputSignals=x,y,v,theta
  Bus Selector2 : BusSelector  OutputSignals=v,theta,vdot,thetadot,curv
  Bus Selector3 : BusSelector  OutputSignals=z1,z2,z3,z4
  Demux : Demux
  Demux1 : Demux  Outputs=2
  Demux2 : Demux  Outputs=2
  Demux3 : Demux
  Derivative : Derivative
  Fcn : Fcn  Expr=u(5)+u(9)*sin(u(8))
  Fcn1 : Fcn  Expr=u(6)-u(9)*cos(u(8))
  Mux : Mux  Inputs=10
  Mux{1..4} (4 alike) : Mux  Inputs=1
  Product{,1..3} (4 alike) : Product
  Signal Conversion : SignalConversion  OverrideOpt=off
  Vector Concatenate : Concatenate  NumInputs=10
  Vector Concatenate1 : Concatenate
  alpha : Subsystem
  disturbance term simplified : Subsystem  Commented=on
  dz3,dz4 calculation : Subsystem
  in parentheses : Subsystem
  invGam : Subsystem
  s : Subsystem
  z1 : Fcn  Expr=u(5)-u(1)+u(9)*sin(u(8))-(r+h*u(3))*cos(u(4))
  z2 : Fcn  Expr=u(6)-u(2)-u(9)*cos(u(8))-(r+h*u(3))*sin(u(4))
  z3 : Fcn  Expr=u(7)*cos(u(8))-u(3)*cos(u(4)+u(10))
  z4 : Fcn  Expr=u(7)*sin(u(8))-u(3)*sin(u(4)+u(10))
  a,w : Outport  VectorParamsAs1DForOutWhenUnconnected=off
  z : Outport  Port=2  VectorParamsAs1DForOutWhenUnconnected=off
  lookahead point : Outport  Port=3  VectorParamsAs1DForOutWhenUnconnected=off
  wires:
  Bus Selector/1 -> Mux/1  "<x>"
  Bus Selector/2 -> Mux/2  "<y>"
  Bus Selector/3 -> Bus Creator1/1, Mux/3  "<v>"
  Bus Selector/4 -> Bus Creator1/2, Mux/4  "<theta>"
  Bus Selector1/1 -> Mux/5  "<x>"
  Bus Selector1/2 -> Mux/6  "<y>"
  Bus Selector1/3 -> Mux/7  "<v>"
  Bus Selector1/4 -> Mux/8  "<theta>"
  Bus Creator/1 -> Signal Conversion/1, [aw]
  state/1 -> alpha/2(state), s/2(state), Bus Selector/1
  state_prec/1 -> alpha/1(state_prec), Bus Selector2/1, s/1(state_prec), Bus Selector1/1
  Mux/1 -> Fcn1/1, Fcn/1, z4/1, z1/1, z2/1, z3/1
  z1/1 -> Bus Creator1/3  "z1"
  z2/1 -> Bus Creator1/4  "z2"
  z3/1 -> Bus Creator1/5  "z3"
  z4/1 -> Bus Creator1/6  "z4"
  alpha/1(alpha) -> Bus Creator1/14, Mux/10  "alpha"
  s/1(s) -> Bus Creator1/13, Mux/9  "s"
  Bus Selector2/1 -> Mux1/1  "<v>"
  Bus Selector2/2 -> Mux2/1  "<theta>"
  Bus Selector2/5 -> Bus Creator1/11, Derivative/1  "<curv>"
  Derivative/1 -> Bus Creator1/12  "curvdot"
  Bus Selector2/4 -> Mux3/1  "<thetadot>"
  Bus Creator1/1 -> invGam/1(In1), dz3,dz4 calculation/2(state), Bus Selector3/1, in parentheses/1(In1)
  invGam/1(invGam) -> Demux/1
  Demux/1 -> Product/1
  in parentheses/1(()) -> Demux1/1
  Demux1/1 -> Product2/2, Product/2
  Demux/2 -> Product1/1
  Product/1 -> Add/1
  Product1/1 -> Add/2
  Demux/3 -> Product2/1
  Demux/4 -> Product3/1
  Demux1/2 -> Product1/2, Product3/2
  Product2/1 -> Add1/1
  Product3/1 -> Add1/2
  Add1/1 -> Bus Creator/2  "w"
  Mux1/1 -> Bus Creator1/7  "v_ref"
  Mux2/1 -> Bus Creator1/8  "theta_ref"
  Bus Selector3/1 -> Vector Concatenate/1  "<z1>"
  Bus Selector3/2 -> Vector Concatenate/2  "<z2>"
  Bus Selector3/3 -> Vector Concatenate/3  "<z3>"
  Bus Selector3/4 -> Vector Concatenate/4  "<z4>"
  Vector Concatenate/1 -> z/1
  Vector Concatenate1/1 -> lookahead point/1
  Fcn/1 -> Vector Concatenate1/1
  Fcn1/1 -> Vector Concatenate1/2
  dz3,dz4 calculation/1(dz3,dz4) -> Demux2/1
  [aw] -> dz3,dz4 calculation/1(a,w)
  Add/1 -> Bus Creator/1  "a"
  Demux2/1 -> Vector Concatenate/5
  Demux2/2 -> Vector Concatenate/6
  Signal Conversion/1 -> a,w/1
  Mux3/1 -> Bus Creator1/10  "thetadot_ref"
  Mux4/1 -> Bus Creator1/9  "vdot_ref"
  Bus Selector2/3 -> Mux4/1  "<vdot>"
  dz3,dz4 calculation/2(Sigma2,Sigma3) -> Demux3/1
  Demux3/1 -> Vector Concatenate/7
  Demux3/2 -> Vector Concatenate/8
  Demux3/3 -> Vector Concatenate/9
  Demux3/4 -> Vector Concatenate/10

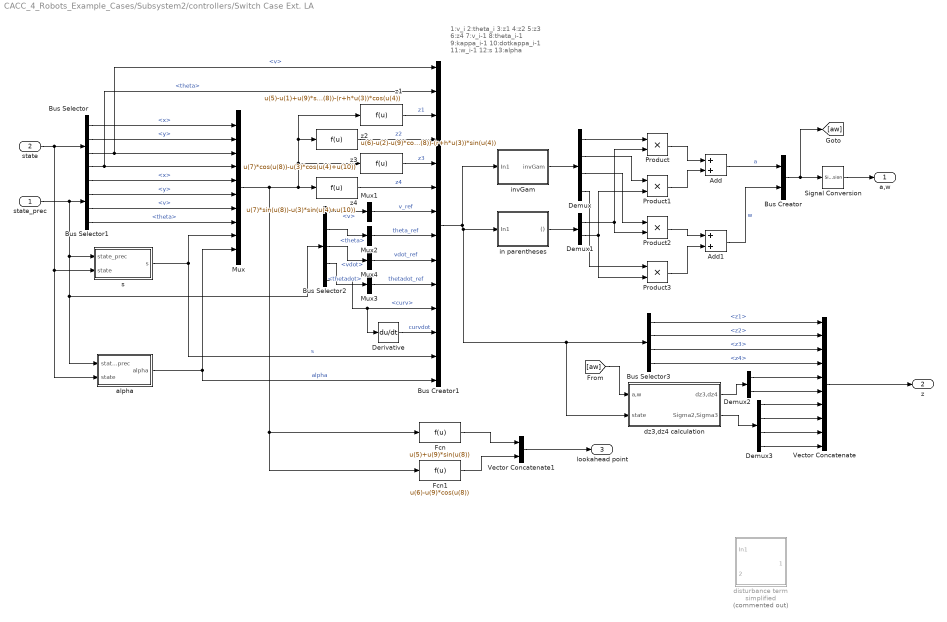
== system CACC_4_Robots_Example_Cases/Subsystem2/controllers/Switch Case Ext. LA ==
  note: 1:v_i
      | 2:theta_i
      | 3:z1
      | 4:z2
      | 5:z3
      | 6:z4
      | 7:v_i-1
      | 8:theta_i-1
      | 9:kappa_i-1
      | 10:dotkappa_i-1
      | 11:w_i-1
      | 12:s
      | 13:alpha
  state_prec : Inport
  state : Inport  Port=2
  Add : Sum
  Add1 : Sum
  Bus Creator : BusCreator  Inputs=2
  Bus Creator1 : BusCreator  Inputs=14
  Bus Selector : BusSelector  OutputSignals=x,y,v,theta
  Bus Selector1 : BusSelector  OutputSignals=x,y,v,theta
  Bus Selector2 : BusSelector  OutputSignals=v,theta,vdot,thetadot,curv
  Bus Selector3 : BusSelector  OutputSignals=z1,z2,z3,z4
  Demux : Demux
  Demux1 : Demux  Outputs=2
  Demux2 : Demux  Outputs=2
  Demux3 : Demux
  Derivative : Derivative
  Fcn : Fcn  Expr=u(5)+u(9)*sin(u(8))
  Fcn1 : Fcn  Expr=u(6)-u(9)*cos(u(8))
  Mux : Mux  Inputs=10
  Mux{1..4} (4 alike) : Mux  Inputs=1
  Product{,1..3} (4 alike) : Product
  Signal Conversion : SignalConversion  OverrideOpt=off
  Vector Concatenate : Concatenate  NumInputs=10
  Vector Concatenate1 : Concatenate
  alpha : Subsystem
  disturbance term simplified : Subsystem  Commented=on
  dz3,dz4 calculation : Subsystem
  in parentheses : Subsystem
  invGam : Subsystem
  s : Subsystem
  z1 : Fcn  Expr=u(5)-u(1)+u(9)*sin(u(8))-(r+h*u(3))*cos(u(4))
  z2 : Fcn  Expr=u(6)-u(2)-u(9)*cos(u(8))-(r+h*u(3))*sin(u(4))
  z3 : Fcn  Expr=u(7)*cos(u(8))-u(3)*cos(u(4)+u(10))
  z4 : Fcn  Expr=u(7)*sin(u(8))-u(3)*sin(u(4)+u(10))
  a,w : Outport  VectorParamsAs1DForOutWhenUnconnected=off
  z : Outport  Port=2  VectorParamsAs1DForOutWhenUnconnected=off
  lookahead point : Outport  Port=3  VectorParamsAs1DForOutWhenUnconnected=off
  wires:
  Bus Selector/1 -> Mux/1  "<x>"
  Bus Selector/2 -> Mux/2  "<y>"
  Bus Selector/3 -> Bus Creator1/1, Mux/3  "<v>"
  Bus Selector/4 -> Bus Creator1/2, Mux/4  "<theta>"
  Bus Selector1/1 -> Mux/5  "<x>"
  Bus Selector1/2 -> Mux/6  "<y>"
  Bus Selector1/3 -> Mux/7  "<v>"
  Bus Selector1/4 -> Mux/8  "<theta>"
  Bus Creator/1 -> Signal Conversion/1, [aw]
  state/1 -> alpha/2(state), s/2(state), Bus Selector/1
  state_prec/1 -> alpha/1(state_prec), Bus Selector2/1, s/1(state_prec), Bus Selector1/1
  Mux/1 -> Fcn1/1, Fcn/1, z4/1, z1/1, z2/1, z3/1
  z1/1 -> Bus Creator1/3  "z1"
  z2/1 -> Bus Creator1/4  "z2"
  z3/1 -> Bus Creator1/5  "z3"
  z4/1 -> Bus Creator1/6  "z4"
  alpha/1(alpha) -> Bus Creator1/14, Mux/10  "alpha"
  s/1(s) -> Bus Creator1/13, Mux/9  "s"
  Bus Selector2/1 -> Mux1/1  "<v>"
  Bus Selector2/2 -> Mux2/1  "<theta>"
  Bus Selector2/5 -> Bus Creator1/11, Derivative/1  "<curv>"
  Derivative/1 -> Bus Creator1/12  "curvdot"
  Bus Selector2/4 -> Mux3/1  "<thetadot>"
  Bus Creator1/1 -> invGam/1(In1), dz3,dz4 calculation/2(state), Bus Selector3/1, in parentheses/1(In1)
  invGam/1(invGam) -> Demux/1
  Demux/1 -> Product/1
  in parentheses/1(()) -> Demux1/1
  Demux1/1 -> Product2/2, Product/2
  Demux/2 -> Product1/1
  Product/1 -> Add/1
  Product1/1 -> Add/2
  Demux/3 -> Product2/1
  Demux/4 -> Product3/1
  Demux1/2 -> Product1/2, Product3/2
  Product2/1 -> Add1/1
  Product3/1 -> Add1/2
  Add1/1 -> Bus Creator/2  "w"
  Mux1/1 -> Bus Creator1/7  "v_ref"
  Mux2/1 -> Bus Creator1/8  "theta_ref"
  Bus Selector3/1 -> Vector Concatenate/1  "<z1>"
  Bus Selector3/2 -> Vector Concatenate/2  "<z2>"
  Bus Selector3/3 -> Vector Concatenate/3  "<z3>"
  Bus Selector3/4 -> Vector Concatenate/4  "<z4>"
  Vector Concatenate/1 -> z/1
  Vector Concatenate1/1 -> lookahead point/1
  Fcn/1 -> Vector Concatenate1/1
  Fcn1/1 -> Vector Concatenate1/2
  dz3,dz4 calculation/1(dz3,dz4) -> Demux2/1
  [aw] -> dz3,dz4 calculation/1(a,w)
  Add/1 -> Bus Creator/1  "a"
  Demux2/1 -> Vector Concatenate/5
  Demux2/2 -> Vector Concatenate/6
  Signal Conversion/1 -> a,w/1
  Mux3/1 -> Bus Creator1/10  "thetadot_ref"
  Mux4/1 -> Bus Creator1/9  "vdot_ref"
  Bus Selector2/3 -> Mux4/1  "<vdot>"
  dz3,dz4 calculation/2(Sigma2,Sigma3) -> Demux3/1
  Demux3/1 -> Vector Concatenate/7
  Demux3/2 -> Vector Concatenate/8
  Demux3/3 -> Vector Concatenate/9
  Demux3/4 -> Vector Concatenate/10

== system CACC_4_Robots_Example_Cases/input reference/circular path small curv/signal: circular path1 ==
  Demux : Demux  Tag=STV Demux  Outputs=2
      settings: DisplayOption=none
  FromWs : FromWorkspace  Tag=STV FromWs  VariableName=tuvar
      SigBuilderData=|
      | common.afterFinalStr = 'Extrapolate'
      | common.sampleTime = 0
      | dataSet.timeRange = [0 40]
      | dataSet.name = 'Group 1'
      | sbobj.Groups.Name = 'Group 1'
      | sbobj.Groups.Signals(1).Name = 'a'
      | sbobj.Groups.Signals(1).XData = [0 40]
      | sbobj.Groups.Signals(1).YData = [0 0]
      | sbobj.Groups.Signals(2).Name = 'omega'
      | sbobj.Groups.Signals(2).XData = [0 6 8 40]
      | sbobj.Groups.Signals(2).YData = [0 0 0.1015 0.1]
      | sbobj.Groups.TimeRange = [0 40]
  a : Outport  Tag=STV Outport  VectorParamsAs1DForOutWhenUnconnected=off
  omega : Outport  Tag=STV Outport  Port=2  VectorParamsAs1DForOutWhenUnconnected=off
  wires:
  FromWs/1 -> Demux/1
  Demux/1 -> a/1
  Demux/2 -> omega/1

== system CACC_4_Robots_Example_Cases/input reference/circular path, varying velocity/signal: circular path1 ==
  Demux : Demux  Tag=STV Demux  Outputs=2
      settings: DisplayOption=none
  FromWs : FromWorkspace  Tag=STV FromWs  VariableName=tuvar
      SigBuilderData=|
      | common.afterFinalStr = 'Extrapolate'
      | common.sampleTime = 0
      | dataSet.timeRange = [0 40]
      | dataSet.name = 'Group 1'
      | sbobj.Groups.Name = 'Group 1'
      | sbobj.Groups.Signals(1).Name = 'a'
      | sbobj.Groups.Signals(1).XData = [0 4 6 8 12 14 16 40]
      | sbobj.Groups.Signals(1).YData = [0 0 0.25 0 0 -0.25 0 0]
      | sbobj.Groups.Signals(2).Name = 'omega'
      | sbobj.Groups.Signals(2).XData = [0 6 8 40]
      | sbobj.Groups.Signals(2).YData = [0 0 0.1 0.1]
      | sbobj.Groups.TimeRange = [0 40]
  a : Outport  Tag=STV Outport  VectorParamsAs1DForOutWhenUnconnected=off
  omega : Outport  Tag=STV Outport  Port=2  VectorParamsAs1DForOutWhenUnconnected=off
  wires:
  FromWs/1 -> Demux/1
  Demux/1 -> a/1
  Demux/2 -> omega/1

== system CACC_4_Robots_Example_Cases/input reference/random path/signal: lane changing ==
  Demux : Demux  Tag=STV Demux  Outputs=2
      settings: DisplayOption=none
  FromWs : FromWorkspace  Tag=STV FromWs  VariableName=tuvar
      SigBuilderData=|
      | common.afterFinalStr = 'Extrapolate'
      | common.sampleTime = 0
      | dataSet.timeRange = [0 40]
      | dataSet.name = 'Group 1'
      | sbobj.Groups.Name = 'Group 1'
      | sbobj.Groups.Signals(1).Name = 'a'
      | sbobj.Groups.Signals(1).XData = [0 40]
      | sbobj.Groups.Signals(1).YData = [0 0]
      | sbobj.Groups.Signals(2).Name = 'omega'
      | sbobj.Groups.Signals(2).XData = [0 4 6 12 14 16 22 24 40]
      | sbobj.Groups.Signals(2).YData = [0 0 0.1 0.1 0 -0.1 -0.1 0 0]
      | sbobj.Groups.TimeRange = [0 40]
  a : Outport  Tag=STV Outport  VectorParamsAs1DForOutWhenUnconnected=off
  omega : Outport  Tag=STV Outport  Port=2  VectorParamsAs1DForOutWhenUnconnected=off
  wires:
  FromWs/1 -> Demux/1
  Demux/1 -> a/1
  Demux/2 -> omega/1

== system CACC_4_Robots_Example_Cases/Subsystem/controllers/Switch Case Ext. LA/alpha ==
  state_prec : Inport
  state : Inport  Port=2
  Bus Selector : BusSelector  OutputSignals=curv
  Bus Selector1 : BusSelector  OutputSignals=v
  Fcn : Fcn  Expr=atan(u(1)*(r+h*u(2)))
  Mux : Mux  Inputs=2
  alpha : Outport  VectorParamsAs1DForOutWhenUnconnected=off
  wires:
  state_prec/1 -> Bus Selector/1
  state/1 -> Bus Selector1/1
  Mux/1 -> Fcn/1
  Bus Selector/1 -> Mux/1  "<curv>"
  Bus Selector1/1 -> Mux/2  "<v>"
  Fcn/1 -> alpha/1

== system CACC_4_Robots_Example_Cases/Subsystem/controllers/Switch Case Ext. LA/disturbance term simplified ==
  In1 : Inport
  (a,w)ref : Inport  Port=2
  Add : Sum  Inputs=-+
  "GamInv " : Subsystem
  H : Subsystem
  H1 : Subsystem
  Product : Product  Inputs=4  Multiplication=Matrix(*)
  Product1 : Product  Multiplication=Matrix(*)
  R(alph) : Subsystem
  beta1 : Subsystem
  dist1,dist2 : Outport  VectorParamsAs1DForOutWhenUnconnected=off
  wires:
  Add/1 -> dist1,dist2/1
  Product/1 -> Add/1
  (a,w)ref/1 -> Product1/2
  H1/1(Out1) -> Product1/1
  beta1/1(Out1) -> Product/4
  "GamInv "/1(GamInv) -> Product/3
  H/1(Out1) -> Product/2
  R(alph)/1(Out1) -> Product/1
  In1/1 -> H/1(In1), R(alph)/1(In1), "GamInv "/1(In1), beta1/1(In1), H1/1(In1)
  Product1/1 -> Add/2
